simulink model "the_last_domaci_kalman"  (R2016a)
settings: Solver=VariableStepAuto  StartTime=0.0  StopTime=100  RelTol=1e-3
values from neighbouring files (symbols this model uses):
  A = [1 a 0]    [main.m]
  Am = [1 alpha1 alpha0]    [main.m]
  B = [b]    [main.m]
  Bm = [alpha0]    [main.m]
  R = [1 r0]    [main.m]
  S = [p1 p0]    [main.m]
  T = [t1 t0]    [main.m]
settings Model: Creator=Vukan  LastModifiedBy=Vukan

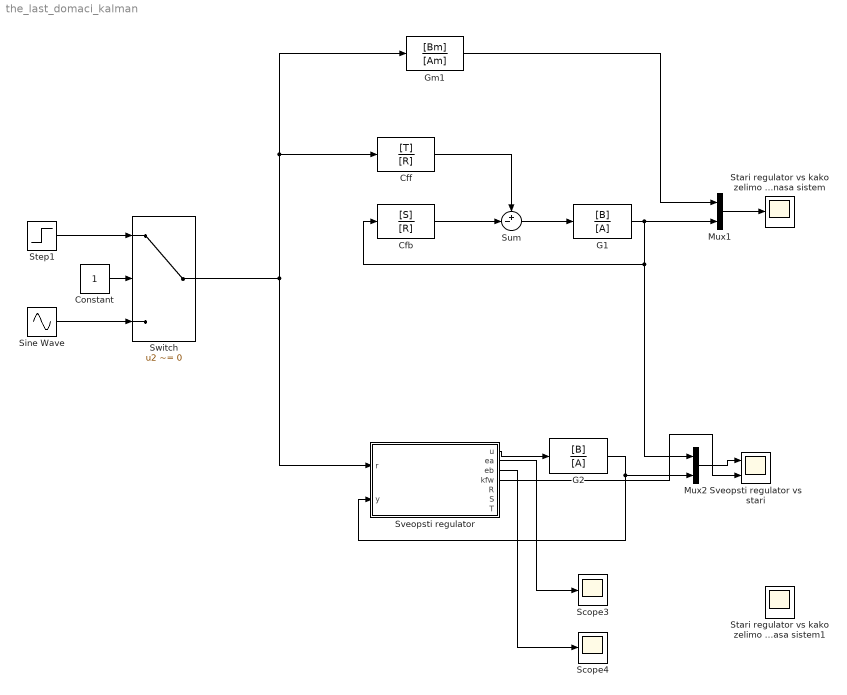
== system the_last_domaci_kalman ==
  Cfb : TransferFcn  Numerator=[S]  Denominator=[R]
  Cff : TransferFcn  Numerator=[T]  Denominator=[R]
  Constant : Constant
  G1 : TransferFcn  Numerator=[B]  Denominator=[A]
  G2 : TransferFcn  Numerator=[B]  Denominator=[A]
  Gm1 : TransferFcn  Numerator=[Bm]  Denominator=[Am]
  Mux1 : Mux  Inputs=2
  Mux2 : Mux  Inputs=2
  Scope3 : Scope
  Scope4 : Scope
  Sine Wave : Sin  SampleTime=0
  Stari regulator vs kako zelimo da se ponasa sistem : Scope
  Stari regulator vs kako zelimo da se ponasa sistem1 : Scope  NumInputPorts=2
  Step1 : Step  SampleTime=0
  Sum : Sum  Inputs=+-|
  Sveopsti regulator : MATLAB Function  TreatAsAtomicUnit=on
  Sveopsti regulator vs stari : Scope  NumInputPorts=2
  Switch : Switch  Criteria=u2 ~= 0
  wires:
  Cfb/1 -> Sum/2
  Cff/1 -> Sum/1
  Sum/1 -> G1/1
  G1/1 -> Mux1/2, Mux2/1, Cfb/1
  Mux1/1 -> Stari regulator vs kako zelimo da se ponasa sistem/1
  Gm1/1 -> Mux1/1
  Mux2/1 -> Sveopsti regulator vs stari/1
  Sveopsti regulator/1(u) -> G2/1
  G2/1 -> Sveopsti regulator/2(y), Mux2/2
  Sveopsti regulator/2(ea) -> Scope3/1
  Sveopsti regulator/3(eb) -> Scope4/1
  Step1/1 -> Switch/1
  Sine Wave/1 -> Switch/3
  Switch/1 -> Cff/1, Gm1/1, Sveopsti regulator/1(r)
  Constant/1 -> Switch/2
  Sveopsti regulator/4(kfw) -> Sveopsti regulator vs stari/2

== matlab function the_last_domaci_kalman/Sveopsti regulator ==
  settings: updateMethod=DISCRETE  sampleTime=Ts
  data: r input; u output; y input; Ts parameter; ea output; eb output; kfw output; R output; S output; T output
function [u, ea, eb, kfw, R, S, T] = sveopsti(r, y, Ts)

% Static variables
persistent yf;
if isempty(yf)
    yf = 0;
end
persistent yp_staro;
if isempty(yp_staro)
    yp_staro = 0;
end
persistent yf1_staro;
if isempty(yf1_staro)
    yf1_staro = 0;
end
persistent rp_staro;
if isempty(rp_staro)
    rp_staro = 0;
end
persistent rf1_staro;
if isempty(rf1_staro)
    rf1_staro = 0;
end
persistent rf;
if isempty(rf)
    rf = 0;
end
persistent P;
if isempty(P)
    P = 10*eye(2);
end
persistent theta;
if isempty(theta)
    theta = [0 0]';
end
persistent u_staro;
if isempty(u_staro)
    u_staro = 0;
end

% ***** Filtering of inputs *****
f_odsecanja = 10;
w_odsecanja = 2*pi*f_odsecanja;
q = w_odsecanja;

% Filtering y
yq = y * q*q;

ypp = yq + yf1_staro*(-q*q) + yp_staro * (-2*q); 
yp_staro = yp_staro + Ts*ypp;
yf1_staro = yf1_staro + Ts*yp_staro;

% Filtering r
rq = r * q*q;

rpp = rq + rf1_staro*(-q*q) + rp_staro * (-2*q); 
rp_staro = rp_staro + Ts*rpp;
rf1_staro = rf1_staro + Ts*rp_staro;

% ***** Recursive Least squares method *****
lambda = 0.9;

% Prepare data
z = ypp;
X = [-yp_staro, u_staro]';

% Update matrix P and estimated parameters in vector theta
P1 = (1/lambda) * (P -   (P*X*X'*P) / (lambda + X'*P*X));
if (X'*P1*X)>0.5*(1-lambda)
    kfw = 1;
    P = P1;
    theta = theta + P*X*(z - X'*theta);
else
    kfw = 0;
end

ea = theta(1);
eb = theta(2);

a = ea;
b = eb;
% a = 2;
% b = 1;
persistent i;
if isempty(i)
    i = 0;
end
i = i + 1;
if i > 100
    % ***** Old part - select parameters and adapt control *****
    ksi = 1;
    w0 = 1;

    alpha0 = w0*w0;
    alpha1 = 2*ksi*w0;
    alpha2 = 3;

    r0 = (alpha1 + alpha2) - a;
    R = [1 r0];

    p0 = alpha0*alpha2 / b;
    p1 = (alpha0 + alpha1*alpha2-a*r0)/b;
    S = [p1 p0];

    t1 = alpha0/b;
    t0 = alpha2*alpha0/b;
    T = [t1 t0];


    % ***** Controller *****
    p = exp(-R(2)*Ts);

    % Feedback part
    yf_staro = yf;
    yf = p * yf_staro + (1-p)*y;
    ufb = (1/R(2)) * ((S(1)/Ts) * (yf - yf_staro) + S(2) * yf);

    % Feedforward part
    rf_staro = rf;
    rf = p * rf_staro + (1-p)*r;
    uff = (1/R(2)) * ((T(1)/Ts) * (rf - rf_staro) + T(2) * rf);

    % Total control signal
    u = uff - ufb;
    u_staro = u;
else
    u = 1;
    u_staro = u;
end
